simulink model "mod_simple2"  (R2014a)
settings: Solver=ode45  StartTime=0.0  StopTime=100.0  RelTol=1e-3
settings Model: Creator=Tanay  LastModifiedBy=Tanay

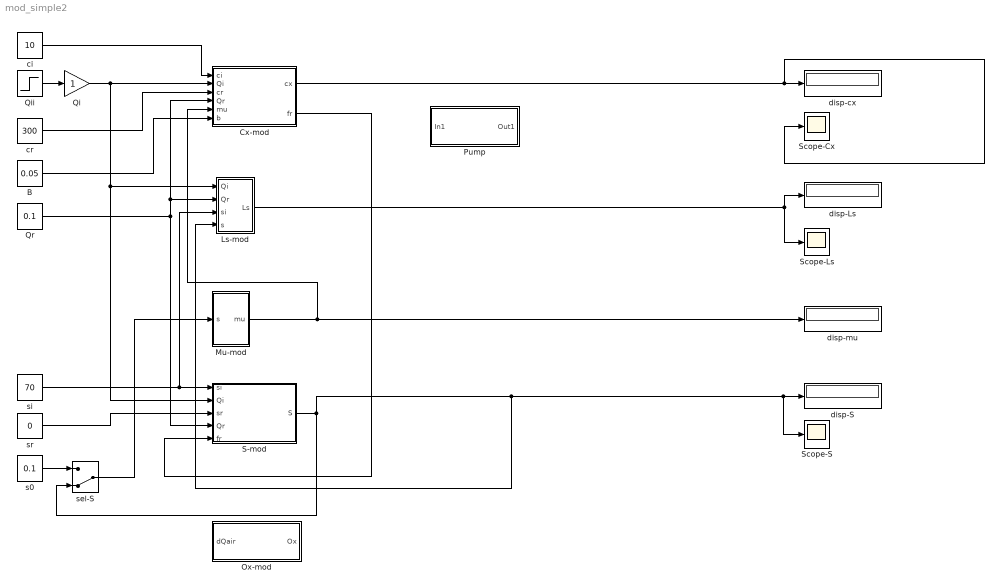
== system mod_simple2 ==
  B : Constant  Value=0.05
  Cx-mod : Subsystem  mask{V=5}
      mask prompts: V "Volume"
  Ls-mod : Subsystem  mask{V=5, Z=0.25}
      mask prompts: V "Volume"
  Mu-mod : Subsystem  mask{mu_max=6, K=5}
      mask prompts: mu_max "Maximum"; K "Dropness"
  Ox-mod : Subsystem  mask{cx_max=10, alpha=1, beta=1}
      mask prompts: cx_max "Oxygen contents"; alpha "Liquefication speed"; beta "Aeration coef."
  Pump : Subsystem
  Qi : Gain
  Qii : Step  SampleTime=0
  Qr : Constant  Value=0.1
  S-mod : Subsystem  mask{V=5, Y=0.01}
      mask prompts: V "Volume"; Y "Regeneration"
  Scope-Cx : Scope
  Scope-Ls : Scope
      settings: SaveName=ScopeData2
  Scope-S : Scope
  ci : Constant  Value=10
  cr : Constant  Value=300
  disp-Ls : Display
  disp-S : Display
  disp-cx : Display
  disp-mu : Display
  s0 : Constant  Value=0.1
  sel-S : ManualSwitch  CurrentSetting=0
  si : Constant  Value=70
  sr : Constant  Value=0
  wires:
  ci/1 -> Cx-mod/1(ci)
  Qii/1 -> Qi/1
  cr/1 -> Cx-mod/3(cr)
  Qr/1 -> Cx-mod/4(Qr), Ls-mod/2(Qr), S-mod/4(Qr)
  B/1 -> Cx-mod/6(b)
  Cx-mod/1(cx) -> Scope-Cx/1, disp-cx/1
  s0/1 -> sel-S/1
  Mu-mod/1(mu) -> Cx-mod/5(mu), disp-mu/1
  S-mod/1(S) -> Ls-mod/4(s), Scope-S/1, disp-S/1, sel-S/2
  si/1 -> S-mod/1(si), Ls-mod/3(si)
  sr/1 -> S-mod/3(sr)
  Cx-mod/2(fr) -> S-mod/5(fr)
  sel-S/1 -> Mu-mod/1(s)
  Qi/1 -> Ls-mod/1(Qi), S-mod/2(Qi), Cx-mod/2(Qi)
  Ls-mod/1(Ls) -> disp-Ls/1, Scope-Ls/1

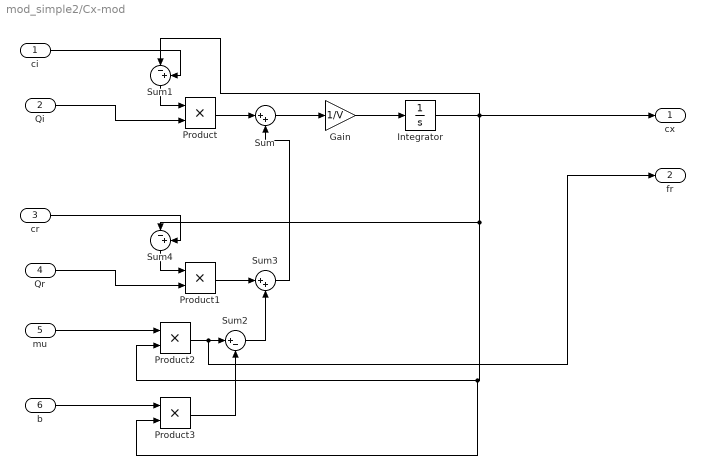
== system mod_simple2/Cx-mod ==
  ci : Inport
  Qi : Inport  Port=2
  cr : Inport  Port=3
  Qr : Inport  Port=4
  mu : Inport  Port=5
  b : Inport  Port=6
  Gain : Gain  Gain=1/V
  Integrator : Integrator
  Product{,1..3} (4 alike) : Product
  Sum : Sum  Inputs=|++
  Sum1 : Sum  Inputs=|-+
  Sum2 : Sum  Inputs=|+-
  Sum3 : Sum  Inputs=|++
  Sum4 : Sum  Inputs=|-+
  cx : Outport
  fr : Outport  Port=2
  wires:
  Sum4/1 -> Product1/1
  Product3/1 -> Sum2/2
  Sum2/1 -> Sum3/2
  Integrator/1 -> cx/1, Product3/2, Product2/2, Sum4/1, Sum1/1
  Product1/1 -> Sum3/1
  Qr/1 -> Product1/2
  cr/1 -> Sum4/2
  Product2/1 -> fr/1, Sum2/1
  b/1 -> Product3/1
  Gain/1 -> Integrator/1
  Sum1/1 -> Product/1
  ci/1 -> Sum1/2
  Sum/1 -> Gain/1
  Qi/1 -> Product/2
  Product/1 -> Sum/1
  mu/1 -> Product2/1
  Sum3/1 -> Sum/2

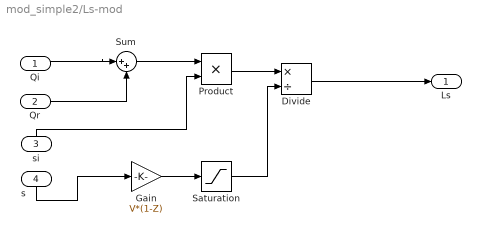
== system mod_simple2/Ls-mod ==
  Qi : Inport
  Qr : Inport  Port=2
  si : Inport  Port=3
  s : Inport  Port=4
  Divide : Product  Inputs=*/
  Gain : Gain  Gain=V*(1-Z)
  Product : Product
  Saturation : Saturate  UpperLimit=1e6  LowerLimit=1e-3
  Sum : Sum  Inputs=|++
  Ls : Outport
  wires:
  Gain/1 -> Saturation/1
  Sum/1 -> Product/1
  Product/1 -> Divide/1
  Qr/1 -> Sum/2
  si/1 -> Product/2
  Divide/1 -> Ls/1
  s/1 -> Gain/1
  Qi/1 -> Sum/1
  Saturation/1 -> Divide/2

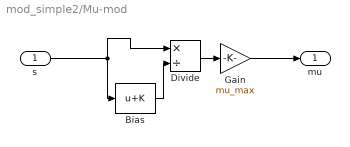
== system mod_simple2/Mu-mod ==
  s : Inport
  Bias : Bias  Bias=K
  Divide : Product  Inputs=*/
  Gain : Gain  Gain=mu_max
  mu : Outport
  wires:
  Gain/1 -> mu/1
  Bias/1 -> Divide/2
  Divide/1 -> Gain/1
  s/1 -> Divide/1, Bias/1

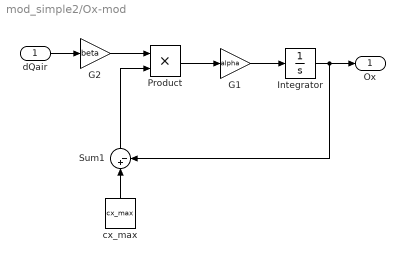
== system mod_simple2/Ox-mod ==
  dQair : Inport
  G1 : Gain  Gain=alpha
  G2 : Gain  Gain=beta
  Integrator : Integrator
  Product : Product
  Sum1 : Sum  Inputs=|+-
  cx_max : Constant  Value=cx_max
  Ox : Outport
  wires:
  Sum1/1 -> Product/2
  cx_max/1 -> Sum1/1
  dQair/1 -> G2/1
  Product/1 -> G1/1
  Integrator/1 -> Sum1/2, Ox/1
  G1/1 -> Integrator/1
  G2/1 -> Product/1

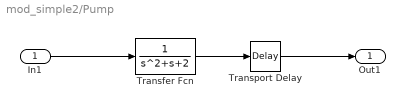
== system mod_simple2/Pump ==
  In1 : Inport
  Transfer Fcn : TransferFcn  Denominator=[1 1 2]
  Transport Delay : TransportDelay
  Out1 : Outport
  wires:
  In1/1 -> Transfer Fcn/1
  Transfer Fcn/1 -> Transport Delay/1
  Transport Delay/1 -> Out1/1

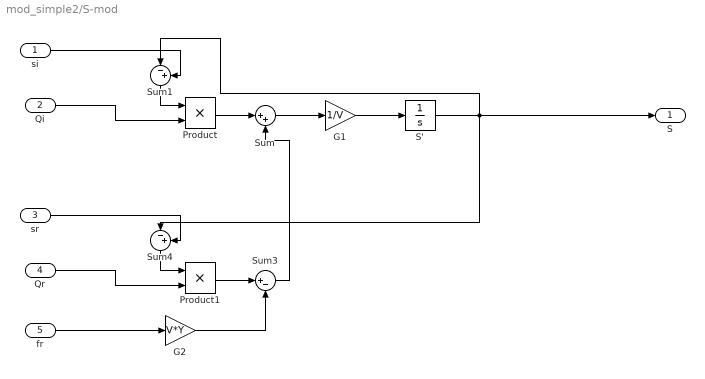
== system mod_simple2/S-mod ==
  si : Inport
  Qi : Inport  Port=2
  sr : Inport  Port=3
  Qr : Inport  Port=4
  fr : Inport  Port=5
  G1 : Gain  Gain=1/V
  G2 : Gain  Gain=V*Y
  Product : Product
  Product1 : Product
  S' : Integrator
  Sum : Sum  Inputs=|++
  Sum1 : Sum  Inputs=|-+
  Sum3 : Sum  Inputs=|+-
  Sum4 : Sum  Inputs=|-+
  S : Outport
  wires:
  Sum4/1 -> Product1/1
  G2/1 -> Sum3/2
  S'/1 -> S/1, Sum4/1, Sum1/1
  Product1/1 -> Sum3/1
  Qr/1 -> Product1/2
  sr/1 -> Sum4/2
  G1/1 -> S'/1
  Sum1/1 -> Product/1
  si/1 -> Sum1/2
  Sum/1 -> G1/1
  Qi/1 -> Product/2
  Product/1 -> Sum/1
  fr/1 -> G2/1
  Sum3/1 -> Sum/2
